simulink model "Gerador_de_dados_remoto"  (R2021b)
settings: Solver=VariableStepAuto  StartTime=0.0  StopTime=50  RelTol=1e-3
settings Model: Creator=duart  LastModifiedBy=duart

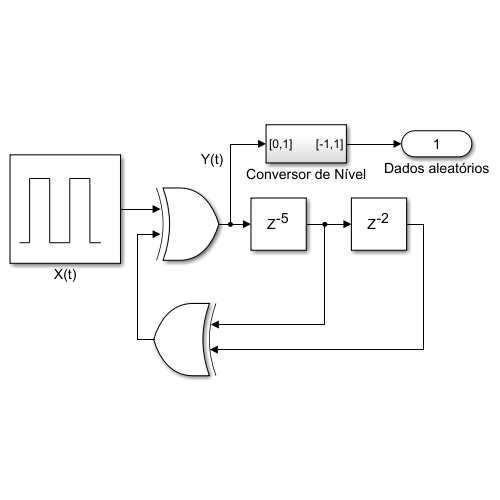
[thumbnail: Simulink's stored preview of the top-level diagram]
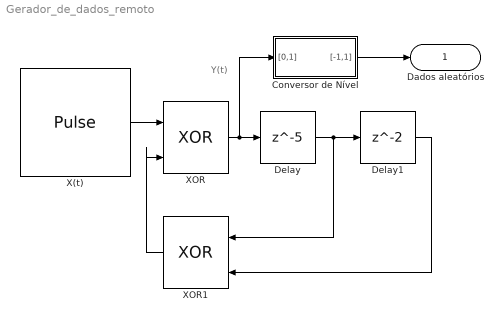
== system Gerador_de_dados_remoto ==
  note: Y(t)
  Conversor de Nível : Subsystem
  Delay : Delay  DelayLength=5  SampleTime=1
  Delay1 : Delay
  X(t) : DiscretePulseGenerator  PulseType=Time based  PulseWidth=50
  XOR : Logic  Operator=XOR  IconShape=distinctive  AllPortsSameDT=off  OutDataTypeStr=boolean
  XOR1 : Logic  Operator=XOR  IconShape=distinctive  AllPortsSameDT=off  OutDataTypeStr=boolean
  Dados aleatórios : Outport
  wires:
  XOR1/1 -> XOR/2
  Delay/1 -> XOR1/1, Delay1/1
  Delay1/1 -> XOR1/2
  XOR/1 -> Conversor de Nível/1("[0,1]"), Delay/1
  Conversor de Nível/1("[-1,1]") -> Dados aleatórios/1
  X(t)/1 -> XOR/1

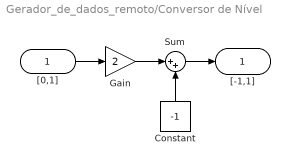
== system Gerador_de_dados_remoto/Conversor de Nível ==
  "[0,1]" : Inport  OutMin=0  OutMax=1
  Constant : Constant  Value=-1
  Gain : Gain  Gain=2
  Sum : Sum  Inputs=|++
  "[-1,1]" : Outport  OutMin=-1  OutMax=1
  wires:
  "[0,1]"/1 -> Gain/1
  Gain/1 -> Sum/1
  Constant/1 -> Sum/2
  Sum/1 -> "[-1,1]"/1
